simulink model "microgrid_y22s_step1"  (R2021b)
settings: Solver=ode45  StartTime=0.0  StopTime=simu.endTime  FixedStep=0.5  MaxStep=simu.maxStepSize  RelTol=1e-3
values from neighbouring files (symbols this model uses):
  A = pi*bladeLength^2    (= 5026.54824574)    [firstinitialization.m]
  rho = 1.2    [firstinitialization.m]
settings Model: Creator=tedbrekken  LastModifiedBy=tedbrekken
settings SolverCC: AlgebraicLoopSolver=TrustRegion
settings DataIOCC: ReturnWorkspaceOutputs=off
settings DebuggingCC: SFMachineParentedDataDiag=warning

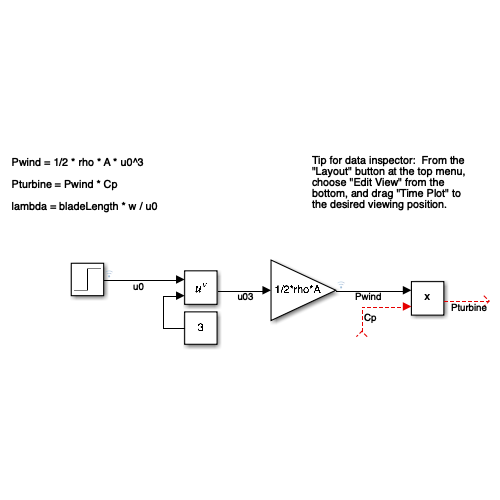
[thumbnail: Simulink's stored preview of the top-level diagram]
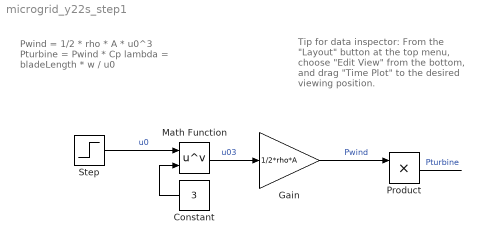
== system microgrid_y22s_step1 ==
  note: Tip for data inspector: From the "Layout" button at the top menu, choose "Edit View" from the bottom, and drag "Time Plot" to the desired viewing position.
  note: Pwind = 1/2 * rho * A * u0^3
      |
      | Pturbine = Pwind * Cp
      |
      | lambda = bladeLength * w / u0
  Constant : Constant  Value=3
  Gain : Gain  Gain=1/2*rho*A
  Math Function : Math  Operator=pow  SaturateOnIntegerOverflow=on
  Product : Product
  Step : Step  Before=5  After=15  SampleTime=0
  wires:
  Math Function/1 -> Gain/1  "u03"
  Gain/1 -> Product/1  "Pwind"
  Step/1 -> Math Function/1  "u0"
  Constant/1 -> Math Function/2
  ? -> Product/2  "Cp"
  Product/1 -> ?  "Pturbine"
